simulink model "lab2task1"  (R2022a)
settings: Solver=VariableStepAuto  StartTime=0.0  StopTime=10.0  RelTol=1e-3
settings Model: Creator=Андрій  LastModifiedBy=Андрій

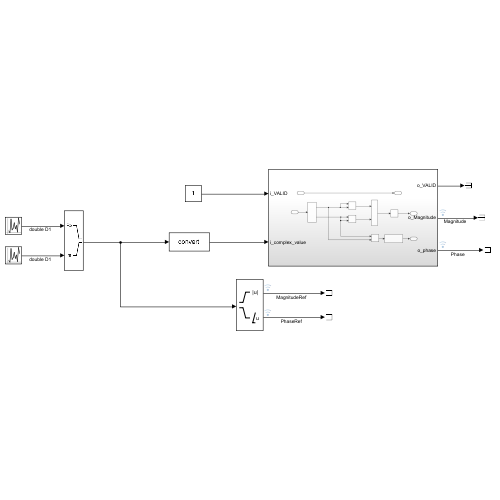
[thumbnail: Simulink's stored preview of the top-level diagram]
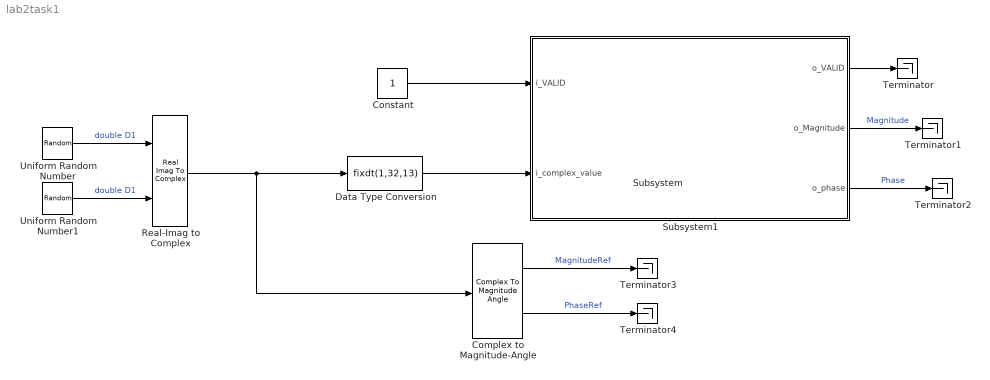
== system lab2task1 ==
  Complex to Magnitude-Angle : ComplexToMagnitudeAngle
  Constant : Constant  OutDataTypeStr=boolean
  Data Type Conversion : DataTypeConversion  OutDataTypeStr=fixdt(1,32,13)  SaturateOnIntegerOverflow=off  RndMeth=Floor
  Real-Imag to Complex : RealImagToComplex
  Subsystem : Subsystem
  Subsystem1 : Subsystem
  Terminator{,1..4} (5 alike) : Terminator
  Uniform Random Number : UniformRandomNumber  Minimum=-2^(19-1)  Maximum=2^(19-1)-1/2^13  Seed=19  SampleTime=1
  Uniform Random Number1 : UniformRandomNumber  Minimum=-2^(19-1)  Maximum=2^(19-1)-1/2^13  Seed=20  SampleTime=1
  wires:
  Uniform Random Number1/1 -> Real-Imag to Complex/2  "double D1"
  Complex to Magnitude-Angle/2 -> Terminator4/1  "PhaseRef"
  Subsystem1/3(o_phase) -> Terminator2/1  "Phase"
  Subsystem1/2(o_Magnitude) -> Terminator1/1  "Magnitude"
  Subsystem1/1(o_VALID) -> Terminator/1
  Real-Imag to Complex/1 -> Data Type Conversion/1, Complex to Magnitude-Angle/1
  Uniform Random Number/1 -> Real-Imag to Complex/1  "double D1"
  Complex to Magnitude-Angle/1 -> Terminator3/1  "MagnitudeRef"
  Data Type Conversion/1 -> Subsystem1/2(i_complex_value)
  Constant/1 -> Subsystem1/1(i_VALID)

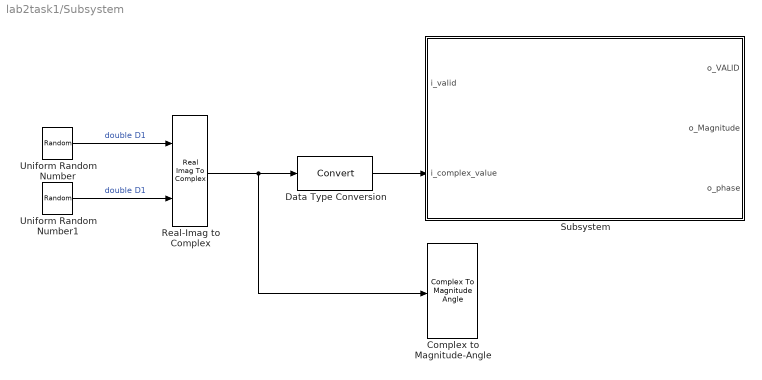
== system lab2task1/Subsystem ==
  Complex to Magnitude-Angle : ComplexToMagnitudeAngle
  Data Type Conversion : DataTypeConversion  SaturateOnIntegerOverflow=off  RndMeth=Floor
  Real-Imag to Complex : RealImagToComplex
  Subsystem : Subsystem
  Uniform Random Number : UniformRandomNumber  SampleTime=0.1
  Uniform Random Number1 : UniformRandomNumber  SampleTime=0.1
  wires:
  Uniform Random Number1/1 -> Real-Imag to Complex/2  "double D1"
  Uniform Random Number/1 -> Real-Imag to Complex/1  "double D1"
  Real-Imag to Complex/1 -> Complex to Magnitude-Angle/1, Data Type Conversion/1
  Data Type Conversion/1 -> Subsystem/2(i_complex_value)

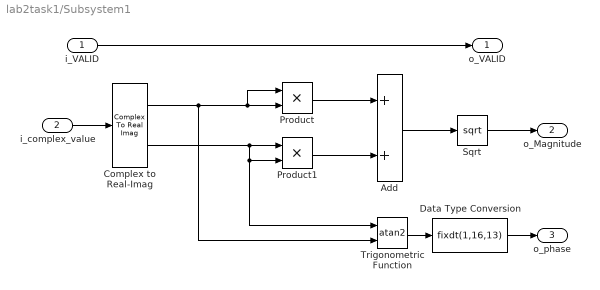
== system lab2task1/Subsystem1 ==
  i_VALID : Inport
  i_complex_value : Inport  Port=2
  Add : Sum
  Complex to Real-Imag : ComplexToRealImag
  Data Type Conversion : DataTypeConversion  OutDataTypeStr=fixdt(1,16,13)  SaturateOnIntegerOverflow=off  RndMeth=Floor
  Product : Product
  Product1 : Product
  Sqrt : Sqrt  OutDataTypeStr=fixdt(1,33,13)
  Trigonometric Function : Trigonometry  Operator=atan2  ApproximationMethod=CORDIC
  o_VALID : Outport
  o_Magnitude : Outport  Port=2
  o_phase : Outport  Port=3
  wires:
  Sqrt/1 -> o_Magnitude/1
  i_VALID/1 -> o_VALID/1
  Complex to Real-Imag/1 -> Trigonometric Function/2, Product/1, Product/2
  Complex to Real-Imag/2 -> Trigonometric Function/1, Product1/2, Product1/1
  Product/1 -> Add/1
  Product1/1 -> Add/2
  Add/1 -> Sqrt/1
  i_complex_value/1 -> Complex to Real-Imag/1
  Trigonometric Function/1 -> Data Type Conversion/1
  Data Type Conversion/1 -> o_phase/1

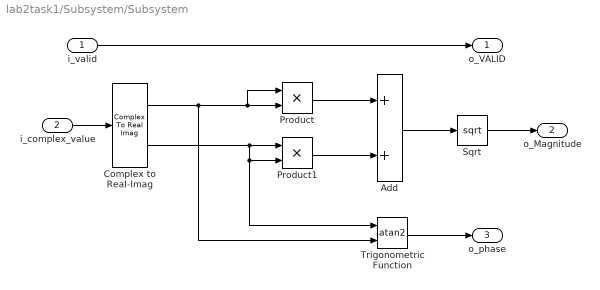
== system lab2task1/Subsystem/Subsystem ==
  i_valid : Inport  OutDataTypeStr=boolean
  i_complex_value : Inport  Port=2  OutDataTypeStr=single
  Add : Sum
  Complex to Real-Imag : ComplexToRealImag
  Product : Product
  Product1 : Product
  Sqrt : Sqrt
  Trigonometric Function : Trigonometry  Operator=atan2
  o_VALID : Outport  OutDataTypeStr=boolean
  o_Magnitude : Outport  Port=2  OutDataTypeStr=single
  o_phase : Outport  Port=3  OutDataTypeStr=single
  wires:
  Sqrt/1 -> o_Magnitude/1
  Trigonometric Function/1 -> o_phase/1
  i_valid/1 -> o_VALID/1
  Complex to Real-Imag/1 -> Trigonometric Function/2, Product/1, Product/2
  Complex to Real-Imag/2 -> Trigonometric Function/1, Product1/2, Product1/1
  Product/1 -> Add/1
  Product1/1 -> Add/2
  Add/1 -> Sqrt/1
  i_complex_value/1 -> Complex to Real-Imag/1
